simulink library "myLibrary"  (R2023b)
settings: Solver=VariableStepAuto  StartTime=0.0  StopTime=10.0  RelTol=1e-3
undefined symbols (not defined in the file): Cac_n1, ctrl1, Da, delta_slk, Discrete, dtha, ee_sli_rtmsupport, FA, gcbh, Ha, Ini, init_DCline, init_IPC, init_line, init_load, init_SG, init_shunt, init_TH, init_trafo, init_user, init_VSC, initMachineBlocks, Ka, Lf, Llkd_pu, Llkq1_pu, magnitude, NET, P, plots_step, q0, Rac_n1, Radd, Rkd_pu, Rkq1_pu, Rload_add, sim_config, sps_rtmsupport, spsSteamTurbineModel, T_DC_NET, T_global, T_IPC, T_load, T_NET, T_SG, T_shunt, T_STATCOM, T_TH, T_trafo, T_user, T_VSC, Ts, tstep, Udiff_a, V1
libraries: spsSeriesRLCBranchLib x120, eeGeneralControl x83, $bdroot x78, spsCurrentMeasurementLib x53, spsParallelRLCBranchLib x39, spsVoltageMeasurementLib x37, spsControlledVoltageSourceLib x30, simulink x29, spsFirstOrderFilterLib x18, spsMeasurementModel x13, spsThreePhaseVIMeasurementLib x5, dspsigops x4
(part 6 of 16)

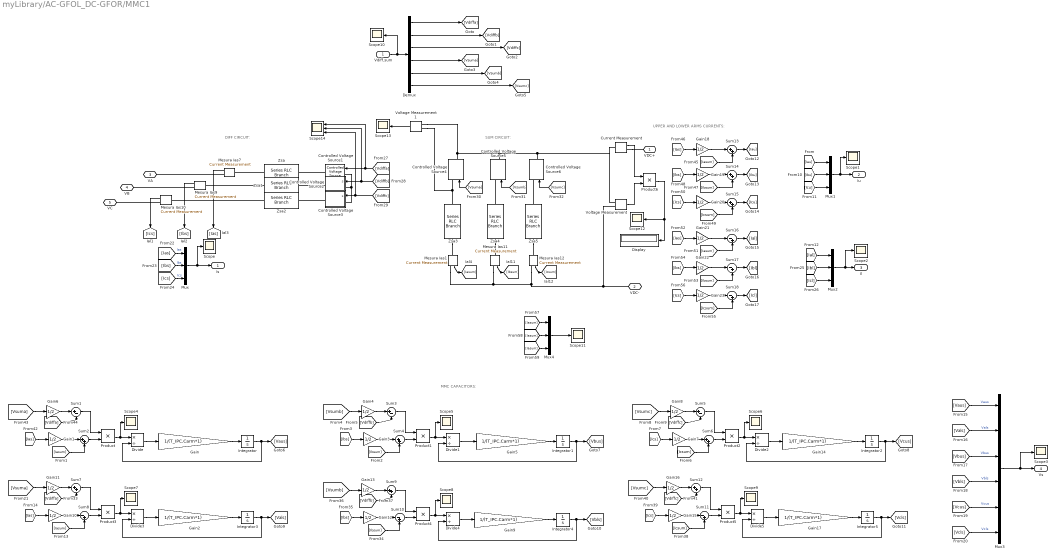
== system myLibrary/AC-GFOL_DC-GFOR/MMC1 ==
  note: DIFF CIRCUIT:
  note: SUM CIRCUIT:
  note: MMC CAPACITORS:
  note: UPPER AND LOWER ARMS CURRENTS:
  Vdiff,sum : Inport
  Controlled Voltage Source1 : spsControlledVoltageSourceLib/Controlled Voltage Source  Initialize=on  Source_Type=AC  Amplitude=initIPC.Udiff_mag  Phase=initIPC.angle_vdiff  Frequency=T_IPC.fb  Measurements=None
  Controlled Voltage Source2 : Subsystem  DialogController=POWERSYS.PowerSysDialog  LoadFcn=sps_rtmsupport('LoadFcn',gcbh);  StartFcn=sps_rtmsupport('StartFcn',gcbh);  StopFcn=sps_rtmsupport('StopFcn',gcbh);  mask(Controlled Voltage Source){Initialize=on, Source_Type=AC, Amplitude=initIPC.Udiff_mag, Phase=initIPC.angle_vdiff-120, Frequency=T_IPC.fb, Measurements=None}
      mask prompts: Source_Type "Source type"; Amplitude "Initial amplitude (V):"; Phase "Initial phase (deg):"; Frequency "Initial frequency (Hz):"
      mask help:
      | Converts the Simulink input signal into an equivalent voltage source. The generated voltage is driven by the input signal of the block.
      |
      | You can initialize your circuit with a specific AC or DC voltage. If you want to start the simulation in steady-state, the block input must be connected to a signal starting as a sinusoidal or DC waveform corresponding to the initial values.
      mask init:
      | powericon('psbloadfunction',gcb,'goto','Initialize');
      | powericon('ControlledSourcesCback',gcb);
      | power_initmask();
      settings: LibrarySourceBlock=spsControlledVoltageSourceLib/Controlled Voltage Source  CopyFcn=sps_rtmsupport('CopyFcn',gcbh); powericon('psbloadfunction',gcb,'goto','UpdateGotoTag');  DeleteFcn=sps_rtmsupport('DeleteFcn',gcbh);  UndoDeleteFcn=sps_rtmsupport('UndoDeleteFcn',gcbh);  ModelCloseFcn=sps_rtmsupport('ModelCloseFcn',gcbh);  PreSaveFcn=sps_rtmsupport('PreSaveFcn',gcbh);  PostSaveFcn=sps_rtmsupport('PostSaveFcn',gcbh);  NameChangeFcn=sps_rtmsupport('NameChangeFcn',gcbh);  PreCopyFcn=sps_rtmsupport('PreCopyFcn',gcbh);  OpenFcn=sps_rtmsupport('OpenFcn',gcbh, [1 2 6]);  CloseFcn=sps_rtmsupport('CloseFcn',gcbh);  PreDeleteFcn=sps_rtmsupport('PreDeleteFcn',gcbh);
      mask Help: helpview(psbhelp);
      mask Callback Initialize: powericon('ControlledSourcesCback',gcb);
      mask TypeOptions Source_Type: AC | DC
      mask Callback Source_Type: powericon('ControlledSourcesCback',gcb);
      mask TypeOptions Measurements: None | Voltage
      mask Display: plot(-50,-35,50,50-15,[0,9,18,24,29,30,29,24,18,9,0,-9,-18,-24,-29,-30,-29,-24,-18,-9,0],[30,29,24,18,9,0,-9,-18,-24,-29,-30,-29,-24,-18,-9,0,9,18,24,29,30],[0,9,18,24,29,30,29,24,18,9,0,-9,-18,-24,-29,-30,-29,-24,-18,-9,0]./-2.4,[1 2 3 4 5 6 7 8 9 10 11 12 13 14 15 16 17 18 19 20 21].*1.5-15);
  Controlled Voltage Source3 : Subsystem  DialogController=POWERSYS.PowerSysDialog  LoadFcn=sps_rtmsupport('LoadFcn',gcbh);  StartFcn=sps_rtmsupport('StartFcn',gcbh);  StopFcn=sps_rtmsupport('StopFcn',gcbh);  mask(Controlled Voltage Source){Initialize=on, Source_Type=AC, Amplitude=initIPC.Udiff_mag, Phase=initIPC.angle_vdiff+120, Frequency=T_IPC.fb, Measurements=None}
      mask prompts: Source_Type "Source type"; Amplitude "Initial amplitude (V):"; Phase "Initial phase (deg):"; Frequency "Initial frequency (Hz):"
      mask help:
      | Converts the Simulink input signal into an equivalent voltage source. The generated voltage is driven by the input signal of the block.
      |
      | You can initialize your circuit with a specific AC or DC voltage. If you want to start the simulation in steady-state, the block input must be connected to a signal starting as a sinusoidal or DC waveform corresponding to the initial values.
      mask init:
      | powericon('psbloadfunction',gcb,'goto','Initialize');
      | powericon('ControlledSourcesCback',gcb);
      | power_initmask();
      settings: LibrarySourceBlock=spsControlledVoltageSourceLib/Controlled Voltage Source  CopyFcn=sps_rtmsupport('CopyFcn',gcbh); powericon('psbloadfunction',gcb,'goto','UpdateGotoTag');  DeleteFcn=sps_rtmsupport('DeleteFcn',gcbh);  UndoDeleteFcn=sps_rtmsupport('UndoDeleteFcn',gcbh);  ModelCloseFcn=sps_rtmsupport('ModelCloseFcn',gcbh);  PreSaveFcn=sps_rtmsupport('PreSaveFcn',gcbh);  PostSaveFcn=sps_rtmsupport('PostSaveFcn',gcbh);  NameChangeFcn=sps_rtmsupport('NameChangeFcn',gcbh);  PreCopyFcn=sps_rtmsupport('PreCopyFcn',gcbh);  OpenFcn=sps_rtmsupport('OpenFcn',gcbh, [1 2 6]);  CloseFcn=sps_rtmsupport('CloseFcn',gcbh);  PreDeleteFcn=sps_rtmsupport('PreDeleteFcn',gcbh);
      mask Help: helpview(psbhelp);
      mask Callback Initialize: powericon('ControlledSourcesCback',gcb);
      mask TypeOptions Source_Type: AC | DC
      mask Callback Source_Type: powericon('ControlledSourcesCback',gcb);
      mask TypeOptions Measurements: None | Voltage
      mask Display: plot(-50,-35,50,50-15,[0,9,18,24,29,30,29,24,18,9,0,-9,-18,-24,-29,-30,-29,-24,-18,-9,0],[30,29,24,18,9,0,-9,-18,-24,-29,-30,-29,-24,-18,-9,0,9,18,24,29,30],[0,9,18,24,29,30,29,24,18,9,0,-9,-18,-24,-29,-30,-29,-24,-18,-9,0]./-2.4,[1 2 3 4 5 6 7 8 9 10 11 12 13 14 15 16 17 18 19 20 21].*1.5-15);
  Controlled Voltage Source4 : spsControlledVoltageSourceLib/Controlled Voltage Source  Initialize=on  Source_Type=DC  Amplitude=initIPC.Usuma  Phase=0  Frequency=0  Measurements=None
  Controlled Voltage Source5 : spsControlledVoltageSourceLib/Controlled Voltage Source  Initialize=on  Source_Type=DC  Amplitude=initIPC.Usumb  Phase=angle(Udiff_a)*180/pi  Frequency=60  Measurements=None
  Controlled Voltage Source6 : spsControlledVoltageSourceLib/Controlled Voltage Source  Initialize=on  Source_Type=DC  Amplitude=initIPC.Usumc  Phase=angle(Udiff_a)*180/pi  Frequency=60  Measurements=None
  Current Measurement : spsCurrentMeasurementLib/Current Measurement  PhasorSimulation=off  OutputType=Complex  PSBequivalent=0
  Demux : Demux  Outputs=6
  Display : Display
  Divide{,1..5} (6 alike) : Product  Inputs=*/
  Gain{,2,5,9,14,17} (6 alike) : Gain  Gain=1/(T_IPC.Carm*1)
  Gain{1,3..4,6..8,10..13,15..16,18..23} (18 alike) : Gain  Gain=1/2
  Integrator{,1..5} (6 alike) : Integrator  InitialCondition=1
  Mesura Ias{1,7,9..12} (6 alike) : spsCurrentMeasurementLib/Current Measurement  PhasorSimulation=off  OutputType=Complex  PSBequivalent=0
  Mux{,1..2,4} (4 alike) : Mux  Inputs=3
  Mux3 : Mux  Inputs=6
  Product{,1..6} (7 alike) : Product
  Scope{,1..13} (14 alike) : Scope
  Scope14 : Scope  NumInputPorts=3
  Sum1 : Sum  Inputs=|+-
  Sum{8,10..11,16..18} (6 alike) : Sum  Inputs=|-+
  Sum{2,4,6..7,9,12..15} (9 alike) : Sum  Inputs=|++
  Sum3 : Sum  Inputs=|+-
  Sum5 : Sum  Inputs=|+-
  Voltage Measurement : spsVoltageMeasurementLib/Voltage Measurement  PhasorSimulation=off  OutputType=Complex  PSBequivalent=0
  Voltage Measurement1 : spsVoltageMeasurementLib/Voltage Measurement  PhasorSimulation=off  OutputType=Complex  PSBequivalent=0
  Zsa : spsSeriesRLCBranchLib/Series RLC Branch  LConnTagsString=__new0  RConnTagsString=__new0  BranchType=RL  Resistance=(T_IPC.Rc+T_IPC.Ra/2)/T_IPC.Sbpu_l2g  Inductance=(T_IPC.Lc+T_IPC.La/2)/T_IPC.Sbpu_l2g  SetiL0=on  InitialCurrent=initIPC.Isa*T_IPC.Sbpu_l2g  Capacitance=1e-6  Setx0=off  InitialVoltage=0  Measurements=None
  Zsa1 : spsSeriesRLCBranchLib/Series RLC Branch  LConnTagsString=__new0  RConnTagsString=__new0  BranchType=RL  Resistance=(T_IPC.Rc+T_IPC.Ra/2)/T_IPC.Sbpu_l2g  Inductance=(T_IPC.Lc+T_IPC.La/2)/T_IPC.Sbpu_l2g  SetiL0=on  InitialCurrent=initIPC.Isb*T_IPC.Sbpu_l2g  Capacitance=1e-6  Setx0=off  InitialVoltage=0  Measurements=None
  Zsa2 : spsSeriesRLCBranchLib/Series RLC Branch  LConnTagsString=__new0  RConnTagsString=__new0  BranchType=RL  Resistance=(T_IPC.Rc+T_IPC.Ra/2)/T_IPC.Sbpu_l2g  Inductance=(T_IPC.Lc+T_IPC.La/2)/T_IPC.Sbpu_l2g  SetiL0=on  InitialCurrent=initIPC.Isc*T_IPC.Sbpu_l2g  Capacitance=1e-6  Setx0=off  InitialVoltage=0  Measurements=None
  Zsa3 : spsSeriesRLCBranchLib/Series RLC Branch  LConnTagsString=__new0  RConnTagsString=__new0  BranchType=RL  Resistance=(2*T_IPC.Ra)/T_IPC.Sbpu_l2g  Inductance=(2*T_IPC.La)/T_IPC.Sbpu_l2g  SetiL0=on  InitialCurrent=initIPC.isum0_DC*T_IPC.Sbpu_l2g  Capacitance=1e-6  Setx0=off  InitialVoltage=0  Measurements=None
  Zsa4 : spsSeriesRLCBranchLib/Series RLC Branch  LConnTagsString=__new0  RConnTagsString=__new0  BranchType=RL  Resistance=(2*T_IPC.Ra)/T_IPC.Sbpu_l2g  Inductance=(2*T_IPC.La)/T_IPC.Sbpu_l2g  SetiL0=on  InitialCurrent=initIPC.isum0_DC*T_IPC.Sbpu_l2g  Capacitance=1e-6  Setx0=off  InitialVoltage=0  Measurements=None
  Zsa5 : spsSeriesRLCBranchLib/Series RLC Branch  LConnTagsString=__new0  RConnTagsString=__new0  BranchType=RL  Resistance=(2*T_IPC.Ra)/T_IPC.Sbpu_l2g  Inductance=(2*T_IPC.La)/T_IPC.Sbpu_l2g  SetiL0=on  InitialCurrent=initIPC.isum0_DC*T_IPC.Sbpu_l2g  Capacitance=1e-6  Setx0=off  InitialVoltage=0  Measurements=None
  VDC+ : PMIOPort  Side=Right
  VDC- : PMIOPort  Port=2  Side=Right
  VA : PMIOPort  Port=3  Side=Left
  VB : PMIOPort  Port=4  Side=Left
  VC : PMIOPort  Port=5  Side=Left
  Is : Outport
  Iu : Outport  Port=2
  Il : Outport  Port=3
  Vs : Outport  Port=4
  wires:
  Mux4/1 -> Scope11/1
  [Iasum] -> Mux4/3
  [Iasum] -> Mux4/2
  [Iasum] -> Mux4/1
  Mesura Ias10/1 -> [Ics]
  Mesura Ias7/1 -> [Ias]
  Mesura Ias9/1 -> [Ibs]
  Vdiff,sum/1 -> Demux/1, Scope10/1
  Demux/5 -> [Vsumb]
  Demux/6 -> [Vsumc]
  Demux/1 -> [Vdiffa]
  Demux/3 -> [Vdiffc]
  Demux/2 -> [Vdiffb]
  Demux/4 -> [Vsuma]
  Mux/1 -> Scope/1, Is/1
  [Ics] -> Mux/3  "Ics"
  [Ibs] -> Mux/2  "Ibs"
  [Ias] -> Mux/1  "Ias"
  [Iau] -> Mux1/1
  [Ibu] -> Mux1/2
  [Icu] -> Mux1/3
  Mux1/1 -> Scope1/1, Iu/1
  [Ial] -> Mux2/1
  Mux2/1 -> Scope2/1, Il/1
  [Icl] -> Mux2/3
  [Vaus] -> Mux3/1  "Vaus"
  [Vals] -> Mux3/2  "Vals"
  [Vbus] -> Mux3/3  "Vbus"
  [Vbls] -> Mux3/4  "Vbls"
  [Vcus] -> Mux3/5  "Vcus"
  [Vcls] -> Mux3/6  "Vcls"
  Mux3/1 -> Scope3/1, Vs/1
  Sum2/1 -> Product/2
  Product/1 -> Scope4/1, Divide/1
  Divide/1 -> Gain/1
  Gain/1 -> Integrator/1
  Integrator/1 -> [Vaus], Divide/2
  [Vdiffa] -> Scope14/1, Controlled Voltage Source1/1
  [Vdiffb] -> Scope14/2, Controlled Voltage Source2/1(s)
  Mesura Ias1/1 -> [Iasum]
  Mesura Ias11/1 -> [Ibsum]
  Mesura Ias12/1 -> [Icsum]
  [Vsuma] -> Controlled Voltage Source4/1
  [Vsumb] -> Controlled Voltage Source5/1
  [Vsumc] -> Controlled Voltage Source6/1
  Gain6/1 -> Sum1/1
  [Vdiffa] -> Sum1/2
  [Iasum] -> Sum2/2
  Gain1/1 -> Sum2/1
  [Ias] -> Gain1/1
  [Vsuma] -> Gain6/1
  Sum1/1 -> Product/1
  Sum3/1 -> Product1/1
  [Vsumb] -> Gain4/1
  [Ibs] -> Gain3/1
  Gain3/1 -> Sum4/1
  [Ibsum] -> Sum4/2
  [Vdiffb] -> Sum3/2
  Gain4/1 -> Sum3/1
  Integrator1/1 -> Divide1/2, [Vbus]
  Gain5/1 -> Integrator1/1
  Divide1/1 -> Gain5/1
  Product1/1 -> Divide1/1, Scope5/1
  Sum4/1 -> Product1/2
  Sum6/1 -> Product2/2
  Product2/1 -> Scope6/1, Divide2/1
  Divide2/1 -> Gain14/1
  Gain14/1 -> Integrator2/1
  Integrator2/1 -> [Vcus], Divide2/2
  Gain8/1 -> Sum5/1
  [Vdiffc] -> Sum5/2
  [Icsum] -> Sum6/2
  Gain7/1 -> Sum6/1
  [Ics] -> Gain7/1
  [Vsumc] -> Gain8/1
  Sum5/1 -> Product2/1
  Sum7/1 -> Product3/1
  [Vsuma] -> Gain11/1
  [Ias] -> Gain10/1
  Gain10/1 -> Sum8/1
  [Iasum] -> Sum8/2
  [Vdiffa] -> Sum7/2
  Gain11/1 -> Sum7/1
  Integrator3/1 -> Divide3/2, [Vals]
  Gain2/1 -> Integrator3/1
  Divide3/1 -> Gain2/1
  Product3/1 -> Divide3/1, Scope7/1
  Sum8/1 -> Product3/2
  Sum10/1 -> Product4/2
  Product4/1 -> Scope8/1, Divide4/1
  Divide4/1 -> Gain9/1
  Gain9/1 -> Integrator4/1
  Integrator4/1 -> [Vbls], Divide4/2
  Gain13/1 -> Sum9/1
  [Vdiffb] -> Sum9/2
  [Ibsum] -> Sum10/2
  Gain12/1 -> Sum10/1
  [Ibs] -> Gain12/1
  [Vsumb] -> Gain13/1
  Sum9/1 -> Product4/1
  Sum12/1 -> Product5/1
  [Vsumc] -> Gain16/1
  [Ics] -> Gain15/1
  Gain15/1 -> Sum11/1
  [Icsum] -> Sum11/2
  [Vdiffc] -> Sum12/2
  Gain16/1 -> Sum12/1
  Integrator5/1 -> Divide5/2, [Vcls]
  Gain17/1 -> Integrator5/1
  Divide5/1 -> Gain17/1
  Product5/1 -> Divide5/1, Scope9/1
  Sum11/1 -> Product5/2
  [Ias] -> Gain18/1
  Gain18/1 -> Sum13/1
  [Iasum] -> Sum13/2
  Sum13/1 -> [Iau]
  Sum14/1 -> [Ibu]
  [Ibsum] -> Sum14/2
  Gain19/1 -> Sum14/1
  [Ibs] -> Gain19/1
  [Ics] -> Gain20/1
  Gain20/1 -> Sum15/1
  [Icsum] -> Sum15/2
  Sum15/1 -> [Icu]
  [Iasum] -> Sum16/2
  [Ias] -> Gain21/1
  Gain21/1 -> Sum16/1
  Sum16/1 -> [Ial]
  Sum17/1 -> [Ibl]
  Gain22/1 -> Sum17/1
  [Ibs] -> Gain22/1
  [Ibsum] -> Sum17/2
  [Icsum] -> Sum18/2
  [Ics] -> Gain23/1
  Gain23/1 -> Sum18/1
  Sum18/1 -> [Icl]
  [Ibl] -> Mux2/2
  Current Measurement/1 -> Product6/1
  Voltage Measurement/1 -> Product6/2
  Product6/1 -> Display/1, Scope12/1
  Voltage Measurement1/1 -> Scope13/1
  [Vdiffc] -> Controlled Voltage Source3/1(s), Scope14/3
  connections:
  Zsa5/RConn1 -- Mesura Ias12/LConn1
  Zsa5/LConn1 -- Controlled Voltage Source6/LConn1
  Zsa4/RConn1 -- Mesura Ias11/LConn1
  Zsa4/LConn1 -- Controlled Voltage Source5/LConn1
  Zsa3/RConn1 -- Mesura Ias1/LConn1
  Zsa3/LConn1 -- Voltage Measurement1/LConn2 -- Controlled Voltage Source4/LConn1
  Mesura Ias7/RConn1 -- VA/RConn1
  Mesura Ias9/RConn1 -- VB/RConn1
  Mesura Ias10/RConn1 -- VC/RConn1
  Zsa/RConn1 -- Mesura Ias7/LConn1
  Zsa1/RConn1 -- Mesura Ias9/LConn1
  Zsa2/RConn1 -- Mesura Ias10/LConn1
  Controlled Voltage Source1/RConn1 -- Zsa/LConn1
  Controlled Voltage Source2/RConn1 -- Zsa1/LConn1
  Controlled Voltage Source3/RConn1 -- Zsa2/LConn1
  Controlled Voltage Source1/LConn1 -- Controlled Voltage Source3/LConn1 -- Controlled Voltage Source2/LConn1
  Controlled Voltage Source6/RConn1 -- Current Measurement/LConn1 -- Voltage Measurement/LConn1 -- Controlled Voltage Source5/RConn1 -- Voltage Measurement1/LConn1 -- Controlled Voltage Source4/RConn1
  Mesura Ias1/RConn1 -- Mesura Ias11/RConn1 -- Mesura Ias12/RConn1 -- Voltage Measurement/LConn2 -- VDC-/RConn1
  Current Measurement/RConn1 -- VDC+/RConn1

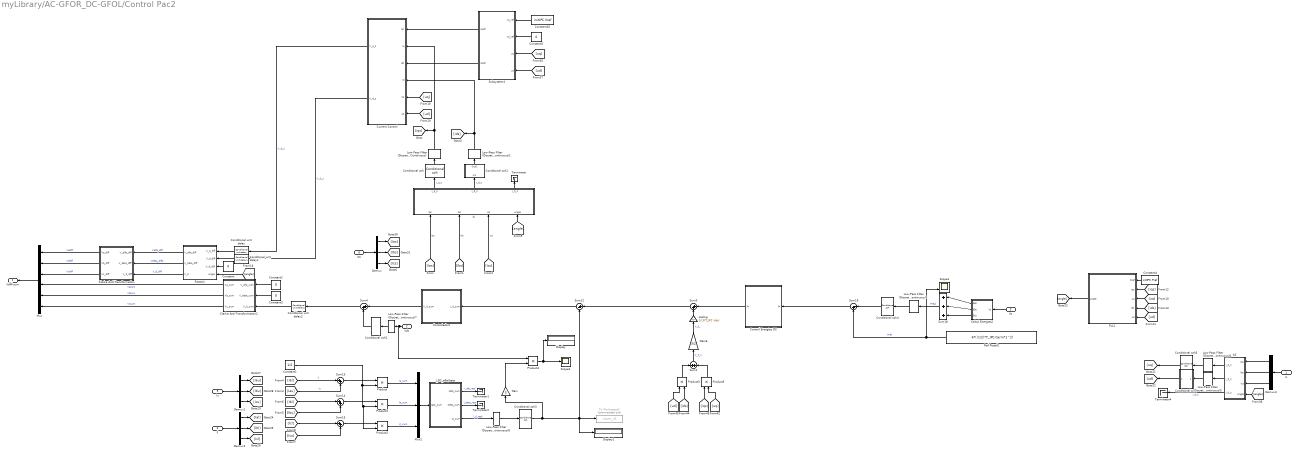
== system myLibrary/AC-GFOR_DC-GFOL/Control Pac2 ==
  U : Inport
  Vdc : Inport  Port=2
  Vs : Inport  Port=3
  Il : Inport  Port=4
  Iu : Inport  Port=5
  Iss : Inport  Port=6
  Calcul Energies2 : Subsystem
  Clarke Anti-Transformation : Subsystem
  Clarke Anti-Transformation2 : Subsystem
  Conditional unit delay : $bdroot/GFOL/Control/Conditional unit delay  SystemSampleTime=-1  VariantActivationTime=update diagram  AllowFlexibleInterface=on  Latency=0  AutoFrameSizeCalculation=off
      link override Constant4: Value=T_IPC.tau_cmd
      link override Unit Delay2: InitialCondition=initIPC.vdiffq  SampleTime=T_IPC.tau_cmd
  Conditional unit delay1 : $bdroot/AC-GFOL_DC-GFOL/Control Pac2/Conditional unit delay1  SystemSampleTime=-1  VariantActivationTime=update diagram  AllowFlexibleInterface=on  Latency=0  AutoFrameSizeCalculation=off
  Conditional unit delay2 : $bdroot/AC-GFOL_DC-GFOL/Control Pac2/Conditional unit delay2  SystemSampleTime=-1  VariantActivationTime=update diagram  AllowFlexibleInterface=on  Latency=0  AutoFrameSizeCalculation=off
  Conditional zoh{,2..5} (5 alike) : $bdroot/AC-GFOL_DC-GFOL/Control Pac2/Conditional zoh  SystemSampleTime=-1  VariantActivationTime=update diagram  AllowFlexibleInterface=on  Latency=0  AutoFrameSizeCalculation=off
  Conditional zoh1 : Subsystem
  Conditional zoh6 : Subsystem
  Constant{,2..3,5} (4 alike) : Constant  Value=0
  Constant1 : Constant  Value=1/2
  Constant10 : Constant  Value=initIPC.Vref
  Constant4 : Constant  Value=initIPC.Pref
  Control Energies DC : Subsystem
  Controladors : Subsystem
  Current Control : Subsystem
  Demux{,1..3} (4 alike) : Demux  Outputs=3
  Display : Display
  Display1 : Display
  Gain : Gain  Gain=3
  Gain6 : Gain  Gain=3/2
  Is : Subsystem
  Is2 : Subsystem
  Low-Pass Filter (Discrete or Continuous) : eeGeneralControl/Low-Pass Filter (Discrete or Continuous)  K=1  T=T_IPC.delay  B=inf  A=-inf  init_option=Specify as parameter  x0=initIPC.idiffq  Ts=0
  Low-Pass Filter (Discrete or Continuous)1 : eeGeneralControl/Low-Pass Filter (Discrete or Continuous)  K=1  T=T_IPC.delay  B=inf  A=-inf  init_option=Specify as parameter  x0=initIPC.idiffd  Ts=0
  Low-Pass Filter (Discrete or Continuous)3 : eeGeneralControl/Low-Pass Filter (Discrete or Continuous)  K=1  T=T_IPC.delay  B=inf  A=-inf  init_option=Specify as parameter  x0=6*((1/2)*T_IPC.Carm*1^2)  Ts=0
  Low-Pass Filter (Discrete or Continuous)4 : eeGeneralControl/Low-Pass Filter (Discrete or Continuous)  K=1  T=T_IPC.delay  B=inf  A=-inf  init_option=Specify as parameter  x0=initIPC.uq  Ts=0
  Low-Pass Filter (Discrete or Continuous)5 : eeGeneralControl/Low-Pass Filter (Discrete or Continuous)  K=1  T=T_IPC.delay  B=inf  A=-inf  init_option=Specify as parameter  x0=initIPC.ud  Ts=0
  Low-Pass Filter (Discrete or Continuous)6 : eeGeneralControl/Low-Pass Filter (Discrete or Continuous)  K=1  T=T_IPC.delay  B=inf  A=-inf  init_option=Specify as parameter  x0=initIPC.isum0_DC  Ts=0
  Low-Pass Filter (Discrete or Continuous)7 : eeGeneralControl/Low-Pass Filter (Discrete or Continuous)  K=1  T=T_IPC.delay  B=inf  A=-inf  init_option=Specify as parameter  x0=initIPC.Vdc  Ts=0
  Mux : Mux  Inputs=6
  Mux2 : Mux  Inputs=3
  PLL1 : Subsystem
  Product{,1..5} (6 alike) : Product
  Ref Ptotal2 : Constant  Value=6*((1/2)*T_IPC.Carm*1^2)
  Rotació : Subsystem
  Scope1 : Scope  NumInputPorts=2
  Scope2 : Scope
  Subsystem4 : Subsystem
  Sum1 : Sum
  Sum12 : Sum  Inputs=|+-
  Sum{3..4,13..15} (5 alike) : Sum  Inputs=|++
  Sum18 : Sum  Inputs=|+++
  Sum19 : Sum  Inputs=|-+
  Terminator{,1..2,4} (4 alike) : Terminator
  To Workspace2 : ToWorkspace  Commented=on  VariableName=isum_n1  SampleTime=plots_step
  l_DC_alfa/beta : Subsystem
  scaling : Gain  Gain=1/(3*T_IPC.Vdc)
  Vdiff-sum : Outport
  wires:
  Product4/1 -> Scope2/1, Display/1
  Gain/1 -> Product4/2
  l_DC_alfa/beta/2(Ibeta_sum) -> Terminator2/1  "I_beta_real"
  l_DC_alfa/beta/1(Ialfa_sum) -> Terminator1/1  "I_afa_real"
  Constant/1 -> Rotació/3(V_0_diff)
  Current Control/2(V_d_s) -> Conditional unit delay1/1  "V_0_s"
  [ids] -> Product3/2
  Product3/1 -> Sum1/1
  Sum3/1 -> Sum12/1
  scaling/1 -> Sum3/2
  [iqs] -> Product5/1
  Control Energies DC/1(Pt') -> Sum3/1
  Product5/1 -> Sum1/2
  Sum1/1 -> Gain6/1  "V_0_s"
  Gain6/1 -> scaling/1  "V_0_"
  [uq] -> Product5/2
  [ud] -> Product3/1
  Subsystem4/1(iqref) -> Current Control/1(Iq*)
  Is2/3(I_0_s) -> Terminator4/1  "I_0_s"
  Sum4/1 -> Conditional unit delay2/1
  Sum19/1 -> Control Energies DC/1(Pt)
  Sum12/1 -> Controladors/1(I_0_sum)
  Controladors/1(V_0_sum) -> Sum4/1
  [ud] -> Current Control/6(ud)
  [uq] -> Current Control/5(uq)
  Current Control/1(V_q_s) -> Conditional unit delay/1  "V_0_s"
  [angle] -> Rotació/4(Angle)
  [angle] -> Is/4(Angle)
  Calcul Energies2/2(Ebt) -> Sum18/2
  Calcul Energies2/3(Ect) -> Sum18/3
  Vs/1 -> Calcul Energies2/1(Vs)
  Iss/1 -> Demux/1
  Demux/3 -> [Ics]
  Demux/2 -> [Ibs]
  Demux/1 -> [Ias]
  Demux3/1 -> Is2/1(Ias)
  Demux3/3 -> Is2/3(Ics)
  U/1 -> Demux3/1
  PLL1/1(Angle) -> [angle]
  [angle] -> Is2/4(Angle)
  Demux3/2 -> Is2/2(Ibs)
  Demux1/2 -> [Ibu]
  Demux2/1 -> [Ial]
  Demux2/3 -> [Icl]
  Il/1 -> Demux2/1
  Demux1/3 -> [Icu]
  Demux1/1 -> [Iau]
  Demux2/2 -> [Ibl]
  Iu/1 -> Demux1/1
  Clarke Anti-Transformation2/3(Vc_sum) -> Mux/6  "Vcsum"
  Sum15/1 -> Product2/1
  [Icu] -> Sum15/2
  [Icl] -> Sum15/1
  Product2/1 -> Mux2/3  "Ic_sum"
  Sum14/1 -> Product1/1
  [Ibu] -> Sum14/2
  [Ibl] -> Sum14/1
  Product1/1 -> Mux2/2  "Ib_sum"
  Constant1/1 -> Product/2, Product1/2, Product2/2
  Sum13/1 -> Product/1
  [Iau] -> Sum13/2  "Iu"
  [Ial] -> Sum13/1  "Il"
  Product/1 -> Mux2/1  "Ia_sum"
  Mux2/1 -> l_DC_alfa/beta/1(Iabc_sum)
  Rotació/2(V_beta_diff) -> Clarke Anti-Transformation/2(V_beta_dfff)  "Vbeta_diffa"
  [Ibs] -> Is/2(Ibs)  "Ibs"
  [Ics] -> Is/3(Ics)  "Ics"
  [Ias] -> Is/1(Ias)  "Ias"
  Rotació/3(V_0) -> Clarke Anti-Transformation/3(V_0_diff)  "V_0_diff"
  Rotació/1(V_alfa_diff) -> Clarke Anti-Transformation/1(V_alfa_diff)  "Valfa_diff"
  Is/1(I_q_s) -> Conditional zoh/1  "I_q_s"
  Is/2(I_d_s) -> Conditional zoh1/1(In1)  "I_d_s"
  Clarke Anti-Transformation/1(Va_diff) -> Mux/1  "Vadiff"
  Clarke Anti-Transformation/2(Vb_diff) -> Mux/2  "Vbdiff"
  Clarke Anti-Transformation/3(Vc_diff) -> Mux/3  "Vcdiff"
  Clarke Anti-Transformation2/2(Vb_sum) -> Mux/5  "Vbsum"
  Clarke Anti-Transformation2/1(Va_sum) -> Mux/4  "Vasum"
  Mux/1 -> Vdiff-sum/1
  Constant3/1 -> Clarke Anti-Transformation2/2(V_beta_sum)
  Constant2/1 -> Clarke Anti-Transformation2/1(V_alfa_sum)
  Calcul Energies2/1(Eat) -> Sum18/1
  Ref Ptotal2/1 -> Sum19/2, Scope1/2  "Pref"
  Low-Pass Filter (Discrete or Continuous)/1 -> [iqs], Current Control/2(Iq)
  Low-Pass Filter (Discrete or Continuous)1/1 -> [ids], Current Control/4(Id)
  Low-Pass Filter (Discrete or Continuous)5/1 -> Conditional zoh6/1(In1)
  Low-Pass Filter (Discrete or Continuous)4/1 -> Conditional zoh5/1
  Low-Pass Filter (Discrete or Continuous)3/1 -> Conditional zoh4/1
  Low-Pass Filter (Discrete or Continuous)7/1 -> Conditional zoh2/1
  Is/3(I_0_s) -> Terminator/1
  Low-Pass Filter (Discrete or Continuous)6/1 -> Conditional zoh3/1
  Constant5/1 -> Subsystem4/2(vd_ref)
  Constant10/1 -> Subsystem4/1(vq_ref)
  [uq] -> Subsystem4/3(vq)
  [ud] -> Subsystem4/4(vd)
  Subsystem4/2(idref) -> Current Control/3(Id*)
  [uq] -> PLL1/3(uq)
  [ud] -> PLL1/5(ud)
  [iqs] -> PLL1/2(iqs)
  [ids] -> PLL1/4(ids)
  Constant4/1 -> PLL1/1(Pref)
  Conditional unit delay1/1 -> Rotació/2(V_d_diff)
  Conditional unit delay/1 -> Rotació/1(V_q_diff)
  Conditional zoh/1 -> Low-Pass Filter (Discrete or Continuous)/1
  Conditional zoh1/1(Out1) -> Low-Pass Filter (Discrete or Continuous)1/1
  Conditional unit delay2/1 -> Clarke Anti-Transformation2/3(V_0_sum)
  Vdc/1 -> Product4/1, Low-Pass Filter (Discrete or Continuous)7/1
  Conditional zoh2/1 -> Sum4/2
  Conditional zoh3/1 -> Sum12/2, To Workspace2/1, Display1/1, Gain/1
  l_DC_alfa/beta/3(I0_sum) -> Low-Pass Filter (Discrete or Continuous)6/1  "I_0_real"
  Is2/1(I_q_s) -> Low-Pass Filter (Discrete or Continuous)4/1
  Is2/2(I_d_s) -> Low-Pass Filter (Discrete or Continuous)5/1
  Conditional zoh6/1(Out1) -> [ud]
  Conditional zoh5/1 -> [uq]
  Sum18/1 -> Low-Pass Filter (Discrete or Continuous)3/1  "Preal"
  Conditional zoh4/1 -> Sum19/1

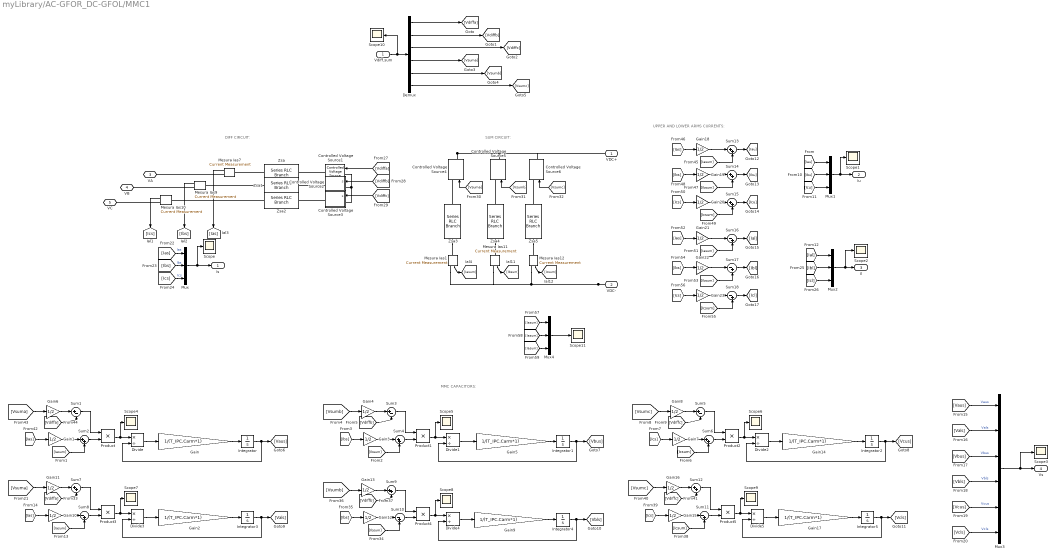
== system myLibrary/AC-GFOR_DC-GFOL/MMC1 ==
  note: UPPER AND LOWER ARMS CURRENTS:
  note: MMC CAPACITORS:
  note: SUM CIRCUIT:
  note: DIFF CIRCUIT:
  Vdiff,sum : Inport
  Controlled Voltage Source1 : spsControlledVoltageSourceLib/Controlled Voltage Source  Initialize=on  Source_Type=AC  Amplitude=initIPC.Udiff_mag  Phase=initIPC.angle_vdiff  Frequency=T_IPC.fb  Measurements=None
  Controlled Voltage Source2 : Subsystem  DialogController=POWERSYS.PowerSysDialog  LoadFcn=sps_rtmsupport('LoadFcn',gcbh);  StartFcn=sps_rtmsupport('StartFcn',gcbh);  StopFcn=sps_rtmsupport('StopFcn',gcbh);  mask(Controlled Voltage Source){Initialize=on, Source_Type=AC, Amplitude=initIPC.Udiff_mag, Phase=initIPC.angle_vdiff-120, Frequency=T_IPC.fb, Measurements=None}
      mask prompts: Source_Type "Source type"; Amplitude "Initial amplitude (V):"; Phase "Initial phase (deg):"; Frequency "Initial frequency (Hz):"
      mask help:
      | Converts the Simulink input signal into an equivalent voltage source. The generated voltage is driven by the input signal of the block.
      |
      | You can initialize your circuit with a specific AC or DC voltage. If you want to start the simulation in steady-state, the block input must be connected to a signal starting as a sinusoidal or DC waveform corresponding to the initial values.
      mask init:
      | powericon('psbloadfunction',gcb,'goto','Initialize');
      | powericon('ControlledSourcesCback',gcb);
      | power_initmask();
      settings: LibrarySourceBlock=spsControlledVoltageSourceLib/Controlled Voltage Source  CopyFcn=sps_rtmsupport('CopyFcn',gcbh); powericon('psbloadfunction',gcb,'goto','UpdateGotoTag');  DeleteFcn=sps_rtmsupport('DeleteFcn',gcbh);  UndoDeleteFcn=sps_rtmsupport('UndoDeleteFcn',gcbh);  ModelCloseFcn=sps_rtmsupport('ModelCloseFcn',gcbh);  PreSaveFcn=sps_rtmsupport('PreSaveFcn',gcbh);  PostSaveFcn=sps_rtmsupport('PostSaveFcn',gcbh);  NameChangeFcn=sps_rtmsupport('NameChangeFcn',gcbh);  PreCopyFcn=sps_rtmsupport('PreCopyFcn',gcbh);  OpenFcn=sps_rtmsupport('OpenFcn',gcbh, [1 2 6]);  CloseFcn=sps_rtmsupport('CloseFcn',gcbh);  PreDeleteFcn=sps_rtmsupport('PreDeleteFcn',gcbh);
      mask Help: helpview(psbhelp);
      mask Callback Initialize: powericon('ControlledSourcesCback',gcb);
      mask TypeOptions Source_Type: AC | DC
      mask Callback Source_Type: powericon('ControlledSourcesCback',gcb);
      mask TypeOptions Measurements: None | Voltage
      mask Display: plot(-50,-35,50,50-15,[0,9,18,24,29,30,29,24,18,9,0,-9,-18,-24,-29,-30,-29,-24,-18,-9,0],[30,29,24,18,9,0,-9,-18,-24,-29,-30,-29,-24,-18,-9,0,9,18,24,29,30],[0,9,18,24,29,30,29,24,18,9,0,-9,-18,-24,-29,-30,-29,-24,-18,-9,0]./-2.4,[1 2 3 4 5 6 7 8 9 10 11 12 13 14 15 16 17 18 19 20 21].*1.5-15);
  Controlled Voltage Source3 : Subsystem  DialogController=POWERSYS.PowerSysDialog  LoadFcn=sps_rtmsupport('LoadFcn',gcbh);  StartFcn=sps_rtmsupport('StartFcn',gcbh);  StopFcn=sps_rtmsupport('StopFcn',gcbh);  mask(Controlled Voltage Source){Initialize=on, Source_Type=AC, Amplitude=initIPC.Udiff_mag, Phase=initIPC.angle_vdiff+120, Frequency=T_IPC.fb, Measurements=None}
      mask prompts: Source_Type "Source type"; Amplitude "Initial amplitude (V):"; Phase "Initial phase (deg):"; Frequency "Initial frequency (Hz):"
      mask help:
      | Converts the Simulink input signal into an equivalent voltage source. The generated voltage is driven by the input signal of the block.
      |
      | You can initialize your circuit with a specific AC or DC voltage. If you want to start the simulation in steady-state, the block input must be connected to a signal starting as a sinusoidal or DC waveform corresponding to the initial values.
      mask init:
      | powericon('psbloadfunction',gcb,'goto','Initialize');
      | powericon('ControlledSourcesCback',gcb);
      | power_initmask();
      settings: LibrarySourceBlock=spsControlledVoltageSourceLib/Controlled Voltage Source  CopyFcn=sps_rtmsupport('CopyFcn',gcbh); powericon('psbloadfunction',gcb,'goto','UpdateGotoTag');  DeleteFcn=sps_rtmsupport('DeleteFcn',gcbh);  UndoDeleteFcn=sps_rtmsupport('UndoDeleteFcn',gcbh);  ModelCloseFcn=sps_rtmsupport('ModelCloseFcn',gcbh);  PreSaveFcn=sps_rtmsupport('PreSaveFcn',gcbh);  PostSaveFcn=sps_rtmsupport('PostSaveFcn',gcbh);  NameChangeFcn=sps_rtmsupport('NameChangeFcn',gcbh);  PreCopyFcn=sps_rtmsupport('PreCopyFcn',gcbh);  OpenFcn=sps_rtmsupport('OpenFcn',gcbh, [1 2 6]);  CloseFcn=sps_rtmsupport('CloseFcn',gcbh);  PreDeleteFcn=sps_rtmsupport('PreDeleteFcn',gcbh);
      mask Help: helpview(psbhelp);
      mask Callback Initialize: powericon('ControlledSourcesCback',gcb);
      mask TypeOptions Source_Type: AC | DC
      mask Callback Source_Type: powericon('ControlledSourcesCback',gcb);
      mask TypeOptions Measurements: None | Voltage
      mask Display: plot(-50,-35,50,50-15,[0,9,18,24,29,30,29,24,18,9,0,-9,-18,-24,-29,-30,-29,-24,-18,-9,0],[30,29,24,18,9,0,-9,-18,-24,-29,-30,-29,-24,-18,-9,0,9,18,24,29,30],[0,9,18,24,29,30,29,24,18,9,0,-9,-18,-24,-29,-30,-29,-24,-18,-9,0]./-2.4,[1 2 3 4 5 6 7 8 9 10 11 12 13 14 15 16 17 18 19 20 21].*1.5-15);
  Controlled Voltage Source4 : spsControlledVoltageSourceLib/Controlled Voltage Source  Initialize=on  Source_Type=DC  Amplitude=initIPC.Usuma  Phase=0  Frequency=0  Measurements=None
  Controlled Voltage Source5 : spsControlledVoltageSourceLib/Controlled Voltage Source  Initialize=on  Source_Type=DC  Amplitude=initIPC.Usumb  Phase=angle(Udiff_a)*180/pi  Frequency=60  Measurements=None
  Controlled Voltage Source6 : spsControlledVoltageSourceLib/Controlled Voltage Source  Initialize=on  Source_Type=DC  Amplitude=initIPC.Usumc  Phase=angle(Udiff_a)*180/pi  Frequency=60  Measurements=None
  Demux : Demux  Outputs=6
  Divide{,1..5} (6 alike) : Product  Inputs=*/
  Gain{,2,5,9,14,17} (6 alike) : Gain  Gain=1/(T_IPC.Carm*1)
  Gain{1,3..4,6..8,10..13,15..16,18..23} (18 alike) : Gain  Gain=1/2
  Integrator{,1..5} (6 alike) : Integrator  InitialCondition=1
  Mesura Ias{1,7,9..12} (6 alike) : spsCurrentMeasurementLib/Current Measurement  PhasorSimulation=off  OutputType=Complex  PSBequivalent=0
  Mux{,1..2,4} (4 alike) : Mux  Inputs=3
  Mux3 : Mux  Inputs=6
  Product{,1..5} (6 alike) : Product
  Scope{,1..11} (12 alike) : Scope
  Sum1 : Sum  Inputs=|+-
  Sum{8,10..11,16..18} (6 alike) : Sum  Inputs=|-+
  Sum{2,4,6..7,9,12..15} (9 alike) : Sum  Inputs=|++
  Sum3 : Sum  Inputs=|+-
  Sum5 : Sum  Inputs=|+-
  Zsa : spsSeriesRLCBranchLib/Series RLC Branch  LConnTagsString=__new0  RConnTagsString=__new0  BranchType=RL  Resistance=(T_IPC.Rc+T_IPC.Ra/2)/T_IPC.Sbpu_l2g  Inductance=(T_IPC.Lc+T_IPC.La/2)/T_IPC.Sbpu_l2g  SetiL0=on  InitialCurrent=initIPC.Isa*T_IPC.Sbpu_l2g  Capacitance=1e-6  Setx0=off  InitialVoltage=0  Measurements=None
  Zsa1 : spsSeriesRLCBranchLib/Series RLC Branch  LConnTagsString=__new0  RConnTagsString=__new0  BranchType=RL  Resistance=(T_IPC.Rc+T_IPC.Ra/2)/T_IPC.Sbpu_l2g  Inductance=(T_IPC.Lc+T_IPC.La/2)/T_IPC.Sbpu_l2g  SetiL0=on  InitialCurrent=initIPC.Isb*T_IPC.Sbpu_l2g  Capacitance=1e-6  Setx0=off  InitialVoltage=0  Measurements=None
  Zsa2 : spsSeriesRLCBranchLib/Series RLC Branch  LConnTagsString=__new0  RConnTagsString=__new0  BranchType=RL  Resistance=(T_IPC.Rc+T_IPC.Ra/2)/T_IPC.Sbpu_l2g  Inductance=(T_IPC.Lc+T_IPC.La/2)/T_IPC.Sbpu_l2g  SetiL0=on  InitialCurrent=initIPC.Isc*T_IPC.Sbpu_l2g  Capacitance=1e-6  Setx0=off  InitialVoltage=0  Measurements=None
  Zsa3 : spsSeriesRLCBranchLib/Series RLC Branch  LConnTagsString=__new0  RConnTagsString=__new0  BranchType=RL  Resistance=(2*T_IPC.Ra)/T_IPC.Sbpu_l2g  Inductance=(2*T_IPC.La)/T_IPC.Sbpu_l2g  SetiL0=on  InitialCurrent=initIPC.isum0_DC*T_IPC.Sbpu_l2g  Capacitance=1e-6  Setx0=off  InitialVoltage=0  Measurements=None
  Zsa4 : spsSeriesRLCBranchLib/Series RLC Branch  LConnTagsString=__new0  RConnTagsString=__new0  BranchType=RL  Resistance=(2*T_IPC.Ra)/T_IPC.Sbpu_l2g  Inductance=(2*T_IPC.La)/T_IPC.Sbpu_l2g  SetiL0=on  InitialCurrent=initIPC.isum0_DC*T_IPC.Sbpu_l2g  Capacitance=1e-6  Setx0=off  InitialVoltage=0  Measurements=None
  Zsa5 : spsSeriesRLCBranchLib/Series RLC Branch  LConnTagsString=__new0  RConnTagsString=__new0  BranchType=RL  Resistance=(2*T_IPC.Ra)/T_IPC.Sbpu_l2g  Inductance=(2*T_IPC.La)/T_IPC.Sbpu_l2g  SetiL0=on  InitialCurrent=initIPC.isum0_DC*T_IPC.Sbpu_l2g  Capacitance=1e-6  Setx0=off  InitialVoltage=0  Measurements=None
  VDC+ : PMIOPort  Side=Right
  VDC- : PMIOPort  Port=2  Side=Right
  VA : PMIOPort  Port=3  Side=Left
  VB : PMIOPort  Port=4  Side=Left
  VC : PMIOPort  Port=5  Side=Left
  Is : Outport
  Iu : Outport  Port=2
  Il : Outport  Port=3
  Vs : Outport  Port=4
  wires:
  [Ibl] -> Mux2/2
  Sum18/1 -> [Icl]
  Gain23/1 -> Sum18/1
  [Ics] -> Gain23/1
  [Icsum] -> Sum18/2
  [Ibsum] -> Sum17/2
  [Ibs] -> Gain22/1
  Gain22/1 -> Sum17/1
  Sum17/1 -> [Ibl]
  Sum16/1 -> [Ial]
  Gain21/1 -> Sum16/1
  [Ias] -> Gain21/1
  [Iasum] -> Sum16/2
  Sum15/1 -> [Icu]
  [Icsum] -> Sum15/2
  Gain20/1 -> Sum15/1
  [Ics] -> Gain20/1
  [Ibs] -> Gain19/1
  Gain19/1 -> Sum14/1
  [Ibsum] -> Sum14/2
  Sum14/1 -> [Ibu]
  Sum13/1 -> [Iau]
  [Iasum] -> Sum13/2
  Gain18/1 -> Sum13/1
  [Ias] -> Gain18/1
  Sum11/1 -> Product5/2
  Product5/1 -> Scope9/1, Divide5/1
  Divide5/1 -> Gain17/1
  Gain17/1 -> Integrator5/1
  Integrator5/1 -> [Vcls], Divide5/2
  Gain16/1 -> Sum12/1
  [Vdiffc] -> Sum12/2
  [Icsum] -> Sum11/2
  Gain15/1 -> Sum11/1
  [Ics] -> Gain15/1
  [Vsumc] -> Gain16/1
  Sum12/1 -> Product5/1
  Sum9/1 -> Product4/1
  [Vsumb] -> Gain13/1
  [Ibs] -> Gain12/1
  Gain12/1 -> Sum10/1
  [Ibsum] -> Sum10/2
  [Vdiffb] -> Sum9/2
  Gain13/1 -> Sum9/1
  Integrator4/1 -> Divide4/2, [Vbls]
  Gain9/1 -> Integrator4/1
  Divide4/1 -> Gain9/1
  Product4/1 -> Divide4/1, Scope8/1
  Sum10/1 -> Product4/2
  Sum8/1 -> Product3/2
  Product3/1 -> Scope7/1, Divide3/1
  Divide3/1 -> Gain2/1
  Gain2/1 -> Integrator3/1
  Integrator3/1 -> [Vals], Divide3/2
  Gain11/1 -> Sum7/1
  [Vdiffa] -> Sum7/2
  [Iasum] -> Sum8/2
  Gain10/1 -> Sum8/1
  [Ias] -> Gain10/1
  [Vsuma] -> Gain11/1
  Sum7/1 -> Product3/1
  Sum5/1 -> Product2/1
  [Vsumc] -> Gain8/1
  [Ics] -> Gain7/1
  Gain7/1 -> Sum6/1
  [Icsum] -> Sum6/2
  [Vdiffc] -> Sum5/2
  Gain8/1 -> Sum5/1
  Integrator2/1 -> Divide2/2, [Vcus]
  Gain14/1 -> Integrator2/1
  Divide2/1 -> Gain14/1
  Product2/1 -> Divide2/1, Scope6/1
  Sum6/1 -> Product2/2
  Sum4/1 -> Product1/2
  Product1/1 -> Scope5/1, Divide1/1
  Divide1/1 -> Gain5/1
  Gain5/1 -> Integrator1/1
  Integrator1/1 -> [Vbus], Divide1/2
  Gain4/1 -> Sum3/1
  [Vdiffb] -> Sum3/2
  [Ibsum] -> Sum4/2
  Gain3/1 -> Sum4/1
  [Ibs] -> Gain3/1
  [Vsumb] -> Gain4/1
  Sum3/1 -> Product1/1
  Sum1/1 -> Product/1
  [Vsuma] -> Gain6/1
  [Ias] -> Gain1/1
  Gain1/1 -> Sum2/1
  [Iasum] -> Sum2/2
  [Vdiffa] -> Sum1/2
  Gain6/1 -> Sum1/1
  [Vsumc] -> Controlled Voltage Source6/1
  [Vsumb] -> Controlled Voltage Source5/1
  [Vsuma] -> Controlled Voltage Source4/1
  Mesura Ias12/1 -> [Icsum]
  Mesura Ias11/1 -> [Ibsum]
  Mesura Ias1/1 -> [Iasum]
  [Vdiffc] -> Controlled Voltage Source3/1(s)
  [Vdiffb] -> Controlled Voltage Source2/1(s)
  [Vdiffa] -> Controlled Voltage Source1/1
  Integrator/1 -> Divide/2, [Vaus]
  Gain/1 -> Integrator/1
  Divide/1 -> Gain/1
  Product/1 -> Divide/1, Scope4/1
  Sum2/1 -> Product/2
  Mux3/1 -> Vs/1, Scope3/1
  [Vcls] -> Mux3/6  "Vcls"
  [Vcus] -> Mux3/5  "Vcus"
  [Vbls] -> Mux3/4  "Vbls"
  [Vbus] -> Mux3/3  "Vbus"
  [Vals] -> Mux3/2  "Vals"
  [Vaus] -> Mux3/1  "Vaus"
  [Icl] -> Mux2/3
  Mux2/1 -> Il/1, Scope2/1
  [Ial] -> Mux2/1
  Mux1/1 -> Iu/1, Scope1/1
  [Icu] -> Mux1/3
  [Ibu] -> Mux1/2
  [Iau] -> Mux1/1
  [Ias] -> Mux/1  "Ias"
  [Ibs] -> Mux/2  "Ibs"
  [Ics] -> Mux/3  "Ics"
  Mux/1 -> Is/1, Scope/1
  Demux/4 -> [Vsuma]
  Demux/2 -> [Vdiffb]
  Demux/3 -> [Vdiffc]
  Demux/1 -> [Vdiffa]
  Demux/6 -> [Vsumc]
  Demux/5 -> [Vsumb]
  Vdiff,sum/1 -> Scope10/1, Demux/1
  Mesura Ias9/1 -> [Ibs]
  Mesura Ias7/1 -> [Ias]
  Mesura Ias10/1 -> [Ics]
  [Iasum] -> Mux4/1
  [Iasum] -> Mux4/2
  [Iasum] -> Mux4/3
  Mux4/1 -> Scope11/1
  connections:
  VDC-/RConn1 -- Mesura Ias12/RConn1 -- Mesura Ias11/RConn1 -- Mesura Ias1/RConn1
  Controlled Voltage Source4/RConn1 -- Controlled Voltage Source5/RConn1 -- Controlled Voltage Source6/RConn1 -- VDC+/RConn1
  Controlled Voltage Source2/LConn1 -- Controlled Voltage Source3/LConn1 -- Controlled Voltage Source1/LConn1
  Controlled Voltage Source3/RConn1 -- Zsa2/LConn1
  Controlled Voltage Source2/RConn1 -- Zsa1/LConn1
  Controlled Voltage Source1/RConn1 -- Zsa/LConn1
  Zsa2/RConn1 -- Mesura Ias10/LConn1
  Zsa1/RConn1 -- Mesura Ias9/LConn1
  Zsa/RConn1 -- Mesura Ias7/LConn1
  Mesura Ias10/RConn1 -- VC/RConn1
  Mesura Ias9/RConn1 -- VB/RConn1
  Mesura Ias7/RConn1 -- VA/RConn1
  Zsa3/LConn1 -- Controlled Voltage Source4/LConn1
  Zsa3/RConn1 -- Mesura Ias1/LConn1
  Zsa4/LConn1 -- Controlled Voltage Source5/LConn1
  Zsa4/RConn1 -- Mesura Ias11/LConn1
  Zsa5/LConn1 -- Controlled Voltage Source6/LConn1
  Zsa5/RConn1 -- Mesura Ias12/LConn1

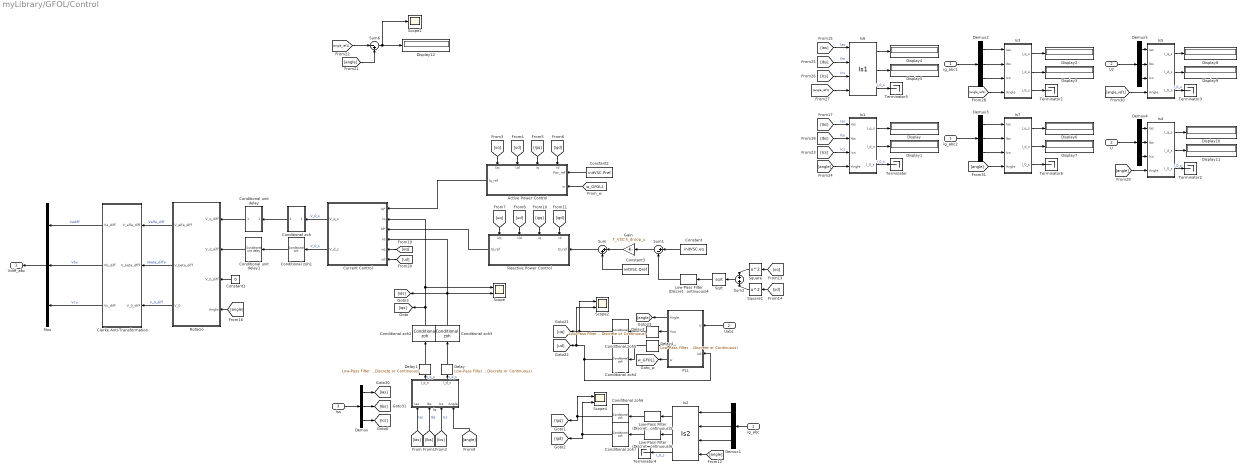
== system myLibrary/GFOL/Control ==
  ig_abc : Inport
  U : Inport  Port=2
  Iss : Inport  Port=3
  Active Power Control : Subsystem
      settings: PortSchema="{\"entries\":[{\"content\":{\"sides\":[{\"content\":{\"connectorIds\":[\"In1\",\"In2\"]},\"type\":\"ConnectorPlacement.EquallySpacedRectSide\",\"uuid\":\"78fe08fc-97ab-4d3f-ad1e-a4935a540f0d\"},{\"content\":{\"connectorIds\":[\"Out1\"],\"side\":\"RIGHT\"},\"type\":\"ConnectorPlacement.EquallySpacedRectSide\",\"uuid\":\"fec6fd50-7083-47ad-a120-ce0b4b3eb939\"},{\"content\":{\"connectorIds\":[\"In3\",\"In4\",\"In5\",\"In6\"],\"side\":\"TOP\"},\"type\":\"ConnectorPlacement.EquallySpacedRectSide\",\"uuid\":\"cab1bf13-1988-4815-ae0e-163353411583\"}]},\"type\":\"ConnectorPlacement.EquallySpacedConnector\",\"uuid\":\"1108cbfd-0203-4acc-b5d3-05af7402b6e2\"}],\"packageUris\":[\"http://schema.mathworks.com/mf0/Connector/R2020b\"],\"version\":\"1.0\"}"
  Clarke Anti-Transformation : Subsystem
  Conditional unit delay : Subsystem
  Conditional unit delay1 : $bdroot/GFOL/Control/Conditional unit delay  SystemSampleTime=-1  VariantActivationTime=update diagram  AllowFlexibleInterface=on  Latency=0  AutoFrameSizeCalculation=off
      link override Unit Delay2: InitialCondition=initVSC.vdiffd
  Conditional zoh : Subsystem
  Conditional zoh{1..7} (7 alike) : $bdroot/GFOL/Control/Conditional zoh  SystemSampleTime=-1  VariantActivationTime=update diagram  AllowFlexibleInterface=on  Latency=0  AutoFrameSizeCalculation=off
  Constant : Constant  Value=initVSC.uq
  Constant1 : Constant  Value=0
  Constant2 : Constant  Value=initVSC.Pref
  Constant3 : Constant  Value=initVSC.Qref
  Current Control : Subsystem
  Delay : eeGeneralControl/Low-Pass Filter (Discrete or Continuous)  K=1  T=T_VSC.tau_md  B=inf  A=-inf  init_option=Specify as parameter  x0=initVSC.idiffd  Ts=0
  Delay1 : eeGeneralControl/Low-Pass Filter (Discrete or Continuous)  K=1  T=T_VSC.tau_md  B=inf  A=-inf  init_option=Specify as parameter  x0=initVSC.idiffq  Ts=0
  Delay3 : eeGeneralControl/Low-Pass Filter (Discrete or Continuous)  K=1  T=T_VSC.tau_md  B=inf  A=-inf  init_option=Specify as parameter  x0=initVSC.uq  Ts=0
  Delay4 : eeGeneralControl/Low-Pass Filter (Discrete or Continuous)  K=1  T=T_VSC.tau_md  B=inf  A=-inf  init_option=Specify as parameter  x0=initVSC.ud  Ts=0
  Demux{,1..5} (6 alike) : Demux  Outputs=3
  Display{,1..12} (13 alike) : Display
  Gain : Gain  Gain=T_VSC.k_droop_u
  Is : Subsystem
  Is1 : Subsystem
  Is2 : $bdroot/GFOR/Control/Is2  SystemSampleTime=-1  VariantActivationTime=update diagram  AllowFlexibleInterface=on  Latency=0  AutoFrameSizeCalculation=off
  Is3 : Subsystem
  Is4 : Subsystem
  Is5 : Subsystem
  Is6 : $bdroot/GFOL/Control/Is1  SystemSampleTime=-1  VariantActivationTime=update diagram  AllowFlexibleInterface=on  Latency=0  AutoFrameSizeCalculation=off
  Is7 : Subsystem
  Low-Pass Filter (Discrete or Continuous)4 : eeGeneralControl/Low-Pass Filter (Discrete or Continuous)  K=1  T=T_VSC.tau_droop_u  B=inf  A=-inf  init_option=Specify as parameter  x0=initVSC.uq  Ts=-1
  Low-Pass Filter (Discrete or Continuous)5 : eeGeneralControl/Low-Pass Filter (Discrete or Continuous)  K=1  T=T_VSC.tau_md  B=inf  A=-inf  init_option=Specify as parameter  x0=initVSC.igq  Ts=0
  Low-Pass Filter (Discrete or Continuous)6 : eeGeneralControl/Low-Pass Filter (Discrete or Continuous)  K=1  T=T_VSC.tau_md  B=inf  A=-inf  init_option=Specify as parameter  x0=initVSC.igd  Ts=0
  Mux : Mux  Inputs=3
  PLL : Subsystem
  Reactive Power Control : Subsystem
      settings: PortSchema="{\"entries\":[{\"content\":{\"sides\":[{\"content\":{\"connectorIds\":[\"In1\"]},\"type\":\"ConnectorPlacement.EquallySpacedRectSide\",\"uuid\":\"78fe08fc-97ab-4d3f-ad1e-a4935a540f0d\"},{\"content\":{\"connectorIds\":[\"Out1\"],\"side\":\"RIGHT\"},\"type\":\"ConnectorPlacement.EquallySpacedRectSide\",\"uuid\":\"fec6fd50-7083-47ad-a120-ce0b4b3eb939\"},{\"content\":{\"connectorIds\":[\"In2\",\"In3\",\"In4\",\"In5\"],\"side\":\"TOP\"},\"type\":\"ConnectorPlacement.EquallySpacedRectSide\",\"uuid\":\"cab1bf13-1988-4815-ae0e-163353411583\"}]},\"type\":\"ConnectorPlacement.EquallySpacedConnector\",\"uuid\":\"1108cbfd-0203-4acc-b5d3-05af7402b6e2\"}],\"packageUris\":[\"http://schema.mathworks.com/mf0/Connector/R2020b\"],\"version\":\"1.0\"}"
  Rotació : Subsystem
  Scope : Scope  NumInputPorts=2
  Scope1 : Scope
  Scope2 : Scope  NumInputPorts=2
  Scope4 : Scope  NumInputPorts=2
  Sqrt : Sqrt
  Square : Math  Operator=square
  Square1 : Math  Operator=square
  Sum : Sum  Inputs=|++
  Sum1 : Sum  Inputs=|+-
  Sum2 : Sum
  Sum6 : Sum  Inputs=|-+
  Terminator{,1..6} (7 alike) : Terminator
  U2 : InportShadow  Port=2
  Uabc : InportShadow  Port=2
  ig_abc1 : InportShadow
  ig_abc2 : InportShadow
  Vdiff_abc : Outport
  tag scope: w_GFOL1=global
  wires:
  Demux1/2 -> Is2/2
  Is2/1 -> Low-Pass Filter (Discrete or Continuous)5/1
  [angle] -> Is2/4
  Is2/2 -> Low-Pass Filter (Discrete or Continuous)6/1
  Is2/3 -> Terminator4/1  "I_0_s"
  Low-Pass Filter (Discrete or Continuous)6/1 -> Conditional zoh7/1
  ig_abc/1 -> Demux1/1
  Demux1/3 -> Is2/3
  Demux1/1 -> Is2/1
  Low-Pass Filter (Discrete or Continuous)5/1 -> Conditional zoh6/1
  Sqrt/1 -> Low-Pass Filter (Discrete or Continuous)4/1
  Delay4/1 -> Conditional zoh4/1
  Delay3/1 -> Conditional zoh5/1
  Constant/1 -> Sum1/1
  Low-Pass Filter (Discrete or Continuous)4/1 -> Sum1/2
  Sum2/1 -> Sqrt/1
  Square1/1 -> Sum2/2
  Square/1 -> Sum2/1
  [ud] -> Square1/1
  [uq] -> Square/1
  Sum1/1 -> Gain/1
  Gain/1 -> Sum/1
  Constant3/1 -> Sum/2
  Sum/1 -> Reactive Power Control/1(Q_ref)
  [w_GFOL1] -> Active Power Control/2(w)
  PLL/4(w) -> [w_GFOL1]
  Is/2(I_d_s) -> Delay/1  "I_d_s"
  Is/1(I_q_s) -> Delay1/1  "I_q_s"
  [Ias] -> Is/1(Ias)  "Ias"
  [Ics] -> Is/3(Ics)  "Ics"
  [Ibs] -> Is/2(Ibs)  "Ibs"
  PLL/1(Angle) -> [angle]
  Uabc/1 -> PLL/1(U)
  Demux/1 -> [Ias]
  Demux/2 -> [Ibs]
  Demux/3 -> [Ics]
  Iss/1 -> Demux/1
  [angle] -> Is/4(Angle)
  [angle] -> Rotació/4(Angle)
  Current Control/1(V_q_s) -> Conditional zoh/1(In1)  "V_0_s"
  Current Control/2(V_d_s) -> Conditional zoh1/1  "V_0_s"
  [uq] -> Current Control/5(uq)
  [ud] -> Current Control/6(ud)
  [angle] -> Sum6/2
  Sum6/1 -> Scope1/1, Display12/1
  [angle_ref1] -> Sum6/1
  [Ias] -> Is1/1(Ias)  "Ias"
  [Ibs] -> Is1/2(Ibs)  "Ibs"
  [Ics] -> Is1/3(Ics)  "Ics"
  [angle] -> Is1/4(Angle)
  [angle_ref1] -> Is3/4(Angle)
  U/1 -> Demux4/1
  Demux4/1 -> Is4/1(Ias)
  Demux4/2 -> Is4/2(Ibs)
  Demux4/3 -> Is4/3(Ics)
  [angle] -> Is4/4(Angle)
  [angle_ref1] -> Is5/4(Angle)
  Demux5/3 -> Is5/3(Ics)
  Demux5/2 -> Is5/2(Ibs)
  Demux5/1 -> Is5/1(Ias)
  U2/1 -> Demux5/1
  Is1/1(I_q_s) -> Display/1
  Is1/2(I_d_s) -> Display1/1
  Is3/1(I_q_s) -> Display2/1
  Is3/2(I_d_s) -> Display3/1
  Is4/1(I_q_s) -> Display10/1
  Is4/2(I_d_s) -> Display11/1
  Is5/1(I_q_s) -> Display8/1
  Is5/2(I_d_s) -> Display9/1
  Is1/3(I_0_s) -> Terminator/1  "I_0_s"
  Is3/3(I_0_s) -> Terminator1/1
  Is4/3(I_0_s) -> Terminator2/1  "I_0_s"
  Is5/3(I_0_s) -> Terminator3/1  "I_0_s"
  Rotació/1(V_alfa_diff) -> Clarke Anti-Transformation/1(V_alfa_diff)  "Valfa_diff"
  Rotació/2(V_beta_diff) -> Clarke Anti-Transformation/2(V_beta_dfff)  "Vbeta_diffa"
  Clarke Anti-Transformation/1(Va_diff) -> Mux/1  "Vadiff"
  Rotació/3(V_0) -> Clarke Anti-Transformation/3(V_0_diff)  "V_0_diff"
  Clarke Anti-Transformation/3(Vc_diff) -> Mux/3  "Vcu"
  Clarke Anti-Transformation/2(Vb_diff) -> Mux/2  "Vbu"
  Mux/1 -> Vdiff_abc/1
  [uq] -> Active Power Control/6(Uq)
  [ud] -> Active Power Control/5(Ud)
  Active Power Control/1(Iq_ref) -> Current Control/1(Iq*)
  Delay/1 -> Conditional zoh3/1
  Delay1/1 -> Conditional zoh2/1
  Constant1/1 -> Rotació/3(V_0_diff)
  PLL/2(Vzq) -> Delay3/1
  PLL/3(Vzd) -> Delay4/1
  [igq] -> Active Power Control/4(iq)
  [igd] -> Active Power Control/3(id)
  Constant2/1 -> Active Power Control/1(Pac_ref)
  [igd] -> Reactive Power Control/2(id)
  [igq] -> Reactive Power Control/3(iq)
  [ud] -> Reactive Power Control/4(Ud)
  [uq] -> Reactive Power Control/5(Uq)
  Reactive Power Control/1(Id_ref) -> Current Control/3(Id*)
  Conditional unit delay/1(Out1) -> Rotació/1(V_q_diff)
  Conditional unit delay1/1 -> Rotació/2(V_d_diff)
  Demux2/1 -> Is3/1(Ias)
  Demux2/2 -> Is3/2(Ibs)
  Demux2/3 -> Is3/3(Ics)
  ig_abc1/1 -> Demux2/1
  Is6/3 -> Terminator5/1  "I_0_s"
  Is6/2 -> Display5/1
  Is6/1 -> Display4/1
  [angle_ref1] -> Is6/4
  [Ics] -> Is6/3  "Ics"
  [Ibs] -> Is6/2  "Ibs"
  [Ias] -> Is6/1  "Ias"
  ig_abc2/1 -> Demux3/1
  Demux3/3 -> Is7/3(Ics)
  Demux3/2 -> Is7/2(Ibs)
  Demux3/1 -> Is7/1(Ias)
  Is7/3(I_0_s) -> Terminator6/1
  Is7/2(I_d_s) -> Display7/1
  Is7/1(I_q_s) -> Display6/1
  [angle] -> Is7/4(Angle)
  Conditional zoh2/1 -> Current Control/2(Iq), Scope/1, [iqs]
  Conditional zoh3/1 -> Scope/2, Current Control/4(Id), [ids]
  Conditional zoh5/1 -> Scope2/1, [uq]
  Conditional zoh4/1 -> Scope2/2, [ud], PLL/2(Ud)
  Conditional zoh6/1 -> [igq], Scope4/1
  Conditional zoh7/1 -> [igd], Scope4/2
  Conditional zoh/1(Out1) -> Conditional unit delay/1(In1)
  Conditional zoh1/1 -> Conditional unit delay1/1

== system myLibrary/GFOL/Electrical ==
  note: DIFF CIRCUIT:
  Vdiff : Inport
  Controlled Voltage Source1 : spsControlledVoltageSourceLib/Controlled Voltage Source  Initialize=on  Source_Type=AC  Amplitude=initVSC.Udiff_mag  Phase=initVSC.angle_vdiff*180/pi  Frequency=T_VSC.fb  Measurements=None
  Controlled Voltage Source2 : spsControlledVoltageSourceLib/Controlled Voltage Source  Initialize=on  Source_Type=AC  Amplitude=initVSC.Udiff_mag  Phase=(initVSC.angle_vdiff -2*pi/3)*180/pi  Frequency=T_VSC.fb  Measurements=None
  Controlled Voltage Source3 : spsControlledVoltageSourceLib/Controlled Voltage Source  Initialize=on  Source_Type=AC  Amplitude=initVSC.Udiff_mag  Phase=(initVSC.angle_vdiff +2*pi/3)*180/pi  Frequency=T_VSC.fb  Measurements=None
  Demux : Demux  Outputs=3
  Mesura Ias10 : spsCurrentMeasurementLib/Current Measurement  PhasorSimulation=off  OutputType=Complex  PSBequivalent=0
  Mesura Ias7 : spsCurrentMeasurementLib/Current Measurement  PhasorSimulation=off  OutputType=Complex  PSBequivalent=0
  Mesura Ias9 : spsCurrentMeasurementLib/Current Measurement  PhasorSimulation=off  OutputType=Complex  PSBequivalent=0
  Mux : Mux  Inputs=3
  Scope : Scope
  Scope10 : Scope  NumInputPorts=3
  Zsa : spsSeriesRLCBranchLib/Series RLC Branch  LConnTagsString=__new0  RConnTagsString=__new0  BranchType=RL  Resistance=initVSC.Rc  Inductance=initVSC.Lc  SetiL0=off  InitialCurrent=initVSC.Isa  Capacitance=1e-6  Setx0=off  InitialVoltage=0  Measurements=None
  Zsa1 : spsSeriesRLCBranchLib/Series RLC Branch  LConnTagsString=__new0  RConnTagsString=__new0  BranchType=RL  Resistance=initVSC.Rc  Inductance=initVSC.Lc  SetiL0=on  InitialCurrent=initVSC.Isb  Capacitance=1e-6  Setx0=off  InitialVoltage=0  Measurements=None
  Zsa2 : spsSeriesRLCBranchLib/Series RLC Branch  LConnTagsString=__new0  RConnTagsString=__new0  BranchType=RL  Resistance=initVSC.Rc  Inductance=initVSC.Lc  SetiL0=on  InitialCurrent=initVSC.Isc  Capacitance=1e-6  Setx0=off  InitialVoltage=0  Measurements=None
  VA : PMIOPort  Side=Left
  VB : PMIOPort  Port=2  Side=Left
  VC : PMIOPort  Port=3  Side=Left
  Is : Outport
  wires:
  Mesura Ias10/1 -> [Ics]
  Mesura Ias7/1 -> [Ias]
  Mesura Ias9/1 -> [Ibs]
  Vdiff/1 -> Demux/1
  Demux/1 -> [Vdiffa]
  Demux/3 -> [Vdiffc]
  Demux/2 -> [Vdiffb]
  Mux/1 -> Scope/1, Is/1
  [Ics] -> Mux/3  "Ics"
  [Ibs] -> Mux/2  "Ibs"
  [Ias] -> Mux/1  "Ias"
  [Vdiffa] -> Controlled Voltage Source1/1, Scope10/1
  [Vdiffb] -> Scope10/2, Controlled Voltage Source2/1
  [Vdiffc] -> Controlled Voltage Source3/1, Scope10/3
  connections:
  Zsa1/LConn1 -- Controlled Voltage Source2/RConn1
  Mesura Ias7/RConn1 -- VA/RConn1
  Mesura Ias9/RConn1 -- VB/RConn1
  Mesura Ias10/RConn1 -- VC/RConn1
  Zsa/RConn1 -- Mesura Ias7/LConn1
  Zsa1/RConn1 -- Mesura Ias9/LConn1
  Zsa2/RConn1 -- Mesura Ias10/LConn1
  Controlled Voltage Source1/RConn1 -- Zsa/LConn1
  Zsa2/LConn1 -- Controlled Voltage Source3/RConn1
  Controlled Voltage Source3/LConn1 -- Controlled Voltage Source1/LConn1 -- Controlled Voltage Source2/LConn1
